simulink model "sl_pursuit"  (R2022a)
settings: Solver=ode45  StartTime=0.0  StopTime=76  FixedStep=0.2  MaxStep=0.1  RelTol=1e-3  EnableMultiTasking=on
StartFcn:
  | % remove the red dashed line draw in StopFcn
  | h = findobj('Tag',  'SL_PURSUIT_PATH');
  | if ~isempty(h)
  |     delete(h)
  | end
StopFcn:
  | % get the waypoints from trajectory block
  | h = getSimulinkBlockHandle([gcs '/trajectory'])
  | path = str2num(get_param(h, 'path'));
  | 
  | % overlay it on the XY scope, tag it so it can be cleaned up in StartFcn
  | set(0, 'ShowHiddenHandles', 'on')
  | fig = findobj('name', 'XY');
  | ax = findobj('type', 'axes');
  | axes(ax);
  | hold on
  | plot(path(:,1), path(:,2), 'Color',  'red', 'LineStyle', '--', 'LineWidth', 2, 'Tag', 'SL_PURSUIT_PATH')
  | grid on
  | hold off
  | set(0, 'ShowHiddenHandles', 'on')
libraries: robotmobilelib x1, roblocks x1, simulink_need_slupdate x1
settings Model: Creator=pic  LastModifiedBy=rpill
settings SolverCC: AlgebraicLoopSolver=TrustRegion  MaxZcPerStep=1
settings DataIOCC: SaveFormat=Array  SignalLoggingSaveFormat=ModelDataLogs  TimeSaveName=t  OutputSaveName=y
settings OptimizationCC: ExpressionDepthLimit=2147483647  LifeSpan=inf
settings DebuggingCC: UnderspecifiedInitializationDetection=Classic  MergeDetectMultiDrivingBlocksExec=none  SolverPrmCheckMsg=warning  FcnCallInpInsideContextMsg=warning  UnconnectedInputMsg=warning  UnconnectedOutputMsg=warning  UnconnectedLineMsg=warning  AllowSymbolicDim=off  StateNameClashWarn=warning  SFUnexpectedBacktrackingDiag=warning  SFNoUnconditionalDefaultTransitionDiag=warning  SFExecutionAtInitializationDiag=none  SFMachineParentedDataDiag=warning  ArithmeticOperatorsInVariantConditions=warning
settings HardwareCC: ProdBitPerPointer=32  ProdBitPerSizeT=32  ProdBitPerPtrDiffT=32  ProdLargestAtomicFloat=None  ProdIntDivRoundTo=Undefined  ProdEndianess=Unspecified  ProdWordSize=32  ProdHWDeviceType=32-bit Generic
settings ModelReferenceCC: PropagateSignalLabelsOutOfModel=off
settings SFSimCC: SimUseLocalCustomCode=off  CustomCodeUndefinedFunction=UseInterfaceOnly
settings RTWCC: RTWUseLocalCustomCode=off  DLArmComputeVersion=19.05
settings CodeAppCC: StateflowObjectComments=on
settings GRTTargetCC: TargetLangStandard=C89/C90 (ANSI)  CombineOutputUpdateFcns=off  GRTInterface=on
settings ConfigComp: CovMetricSettings=dw  CovSaveCumulativeToWorkspaceVar=on  CovSaveSingleToWorkspaceVar=on  CovExternalEMLEnable=off

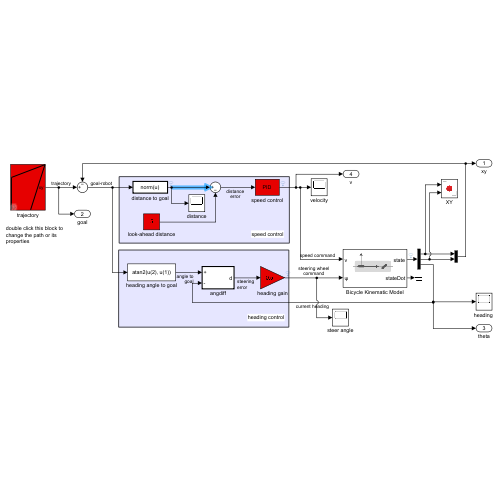
[thumbnail: Simulink's stored preview of the top-level diagram]
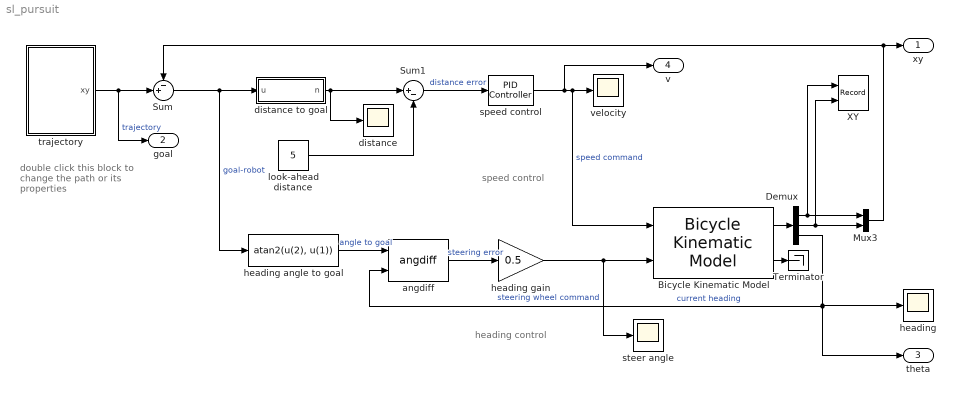
== system sl_pursuit ==
  note: speed control
  note: heading control
  note: double click this block to
      | change the path or its
      | properties
  Bicycle Kinematic Model : robotmobilelib/Bicycle Kinematic Model  VehicleInputs=Vehicle Speed & Steering Angle  WheelBase=1  VehicleSpeedRange=[0 5]  MaxSteeringAngle=0.5  InitialState=[0 0 0]  SimulateUsing=Interpreted execution
      settings: SourceProductBaseCode=RO
  Demux : Demux  Outputs=3
  Mux3 : Mux  Inputs=2
  Sum : Sum  Inputs=-+|
  Sum1 : Sum  Inputs=|+-
  Terminator : Terminator
  XY : Record  FileSettingsInternal="{\"entries\":[{\"content\":{\"excelSettings\":{\"content\":{},\"type\":\"Streamout.ExcelSettings\"}},\"type\":\"Streamout.FileSettingStorage\",\"uuid\":\"1ab6e84b-ba46-4ab6-9ea9-c76159d60a93\"}],\"packageUris\":[\"http://schema.mathworks.com/mf0/streamout_blocks/R2020a\"],\"version\":\"1.0\"}"  Layout=[1 1]  SignalsInternal="{\"entries\":[{\"content\":{\"signals\":[{\"content\":{\"blockPath\":[\"sl_pursuit/XY\"],\"channel\":[],\"dimensions\":[1],\"domain\":\"sl_pursuit/XY\",\"lineColor\":\"#a2142f\",\"plots\":[1],\"port\":1,\"sid\":[],\"signalID\":541,\"signalName\":\"XY Graph:1\"},\"type\":\"RecordBlkView.Signal\",\"uuid\":\"bba33781-1f45-4acc-9c6b-d804efa5f02e\"},{\"content\":{\"blockPath\":[\"sl_pursuit/XY\"],\"channel\":[],\"dimensions\":[1],\"domain\":\"sl_pursuit/XY\",\"lineColor\":\"#139fff\",\"plots\":[1],\"port\":2,\"sid\":[],\"signalID\":544,\"signalName\":\"XY Graph:2\"},\"type\":\"RecordBlkView.Signal\",\"uuid\":\"3768845e-2c8a-4000-8acb-070147153844\"}]},\"type\":\"RecordBlkView.InputSignals\",\"uuid\":\"8d282ecb-477a-4c26-82d2-7eb094f92171\"}],\"packageUris\":[\"http://schema.mathworks.com/mf0/streamout_blocks/R2020a\"],\"version\":\"1.0\"}"  VisualizationBindings="{\"xyplotplugin\":{\"info\":[{\"series\":[{\"bindingParametersList\":[{\"parameter\":\"X-Axis\",\"signalID\":541,\"signalName\":\"XY Graph:1\"},{\"parameter\":\"Y-Axis\",\"signalID\":544,\"signalName\":\"XY Graph:2\"}],\"seriesID\":33980}],\"subplotID\":1}]}}"  CompatibilityTag=XY  st=-1
  angdiff : roblocks/angdiff  SystemSampleTime=-1  VariantActivationTime=update diagram  Latency=0  AutoFrameSizeCalculation=off
  distance : Scope
  distance to goal : MATLAB Function  TreatAsAtomicUnit=on
  "heading " : Scope
  heading angle to goal : Fcn  Expr=atan2(u(2), u(1))
  heading gain : Gain  Gain=0.5
  look-ahead distance : Constant  Value=5
  speed control : simulink_need_slupdate/PID Controller  P=1  I=0.1  D=0
  steer angle : Scope
  trajectory : Subsystem  mask(Trajectory generator){path=|, vaxis=[2.5 2.5], tseg=[], dt=0.1, tacc=0, setsimtime=on}
      mask path=|
      | [  10 10;
      |   10 60;
      |   80 80;
      |   50 10 ]
      mask prompts: vaxis "Axis velocities"; tseg "Segment times"; dt "Sample interval"; tacc "Acceleration time"; setsimtime "Set Simulink simulation time"
      mask help: Generate an n-dimensional trajectory using the Toolbox function mstraj.
      mask init:
      | robot_traj = mstraj(path(2:end,:), vaxis, tseg, path(1,:), dt, tacc);
      | total_time = size(robot_traj,1)*dt;
      | if setsimtime
      |     set_param(gcs, 'StopTime', num2str(total_time));
      | end
      mask Help:
      | The trajectory requires a number of parameters
      | 
      | Path: an MxN matrix that defines a path with M points (start, intermediate, goal) and each point is defined by an N-dimensional vector.
      | 
      | Axis velocities: a 1xM vector that specifies the maximum speed of each motion for each dimension.
      | 
      | Segment times: a 1x(N-1) vector of times to execute each motion segment.
      | 
      | Sample time: a scalar sampling time, the trajectory is computed at discrete times with this separation.
      | 
      | Acceleration time: a scalar giving the period of acceleration at each waypoint, as the motion accelerates from one segment to the next.  Can be zero.
      | 
      | This block sets the Simulink simulation time to the length of the trajectory.
      mask Display: plot(path(:,1), path(:,2))
  velocity : Scope
  xy : Outport  VectorParamsAs1DForOutWhenUnconnected=off
  goal : Outport  Port=2  VectorParamsAs1DForOutWhenUnconnected=off
  theta : Outport  Port=3  VectorParamsAs1DForOutWhenUnconnected=off
  v : Outport  Port=4  VectorParamsAs1DForOutWhenUnconnected=off
  wires:
  Mux3/1 -> Sum/1, xy/1
  Sum/1 -> distance to goal/1(u), heading angle to goal/1  "goal-robot"
  heading angle to goal/1 -> angdiff/1  "angle to goal"
  Demux/3 -> angdiff/2, theta/1, "heading "/1  "current heading"
  angdiff/1 -> heading gain/1  "steering error"
  heading gain/1 -> steer angle/1, Bicycle Kinematic Model/2  "steering wheel command"
  speed control/1 -> Bicycle Kinematic Model/1, velocity/1, v/1  "speed command"
  distance to goal/1(n) -> Sum1/1, distance/1
  trajectory/1(xy) -> goal/1, Sum/2  "trajectory"
  Sum1/1 -> speed control/1  "distance error"
  look-ahead distance/1 -> Sum1/2
  Bicycle Kinematic Model/1 -> Demux/1
  Demux/1 -> XY/1, Mux3/1
  Demux/2 -> XY/2, Mux3/2
  Bicycle Kinematic Model/2 -> Terminator/1

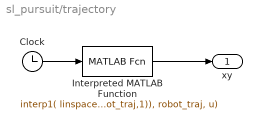
== system sl_pursuit/trajectory ==
  Clock : Clock
  Interpreted MATLAB Function : MATLABFcn  MATLABFcn=interp1( linspace(0, total_time, size(robot_traj,1)), robot_traj, u)
  xy : Outport  VectorParamsAs1DForOutWhenUnconnected=off
  wires:
  Clock/1 -> Interpreted MATLAB Function/1
  Interpreted MATLAB Function/1 -> xy/1

== matlab function sl_pursuit/distance to goal ==
  data: u input; n output
function n = norm(u)

n = norm(u);

end
